simulink model "MassSpringDamperModel"  (R2026a)
settings: Solver=VariableStepAuto  StopTime=Inf  MaxStep=inf  RelTol=1e-6
values from neighbouring files (symbols this model uses):
  b = 1.0    [MassSpringDamperModelData.sldd]    (also in MassSpringDamperModelEventsData.sldd = 3.0)
  k = 100.0    [MassSpringDamperModelData.sldd]    (also in MassSpringDamperModelEventsData.sldd = 128.0)
  m = 10.0    [MassSpringDamperModelData.sldd]    (also in MassSpringDamperModelEventsData.sldd = 2.0)
  x0 = 0.5    [MassSpringDamperModelData.sldd]    (also in MassSpringDamperModelEventsData.sldd = 5.0)
libraries: simulink x1
Description:
  | The van der Pol Equation
  | 
  | This is a simulation of a nonlinear second order system.
settings Model: DataDictionary=MassSpringDamperModelData.sldd  ExtModeAutoUpdateStatusClock=off  Creator=The MathWorks, Inc.  LastModifiedBy=kdeeley
settings DataIOCC: ExternalInput=[]  InitialState=[]  TimeSaveName=t  OutputSaveName=y
settings OptimizationCC: BooleanDataType=off  InitFltsAndDblsToZero=on  BufferReusableBoundary=off
settings DebuggingCC: SaveWithParameterizedLinksMsg=none  SignalResolutionControl=TryResolveAllWithWarning  MultiTaskDSMMsg=warning  MultiTaskCondExecSysMsg=none  BusObjectLabelMismatch=none  PregeneratedLibrarySubsystemCodeDiagnostic=none
settings HardwareCC: ProdHWDeviceType=32-bit Generic  TargetUnknown=on
settings GRTTargetCC: TargetFcnLib=ansi_tfl_tmw.mat  CombineOutputUpdateFcns=off  GRTInterface=on

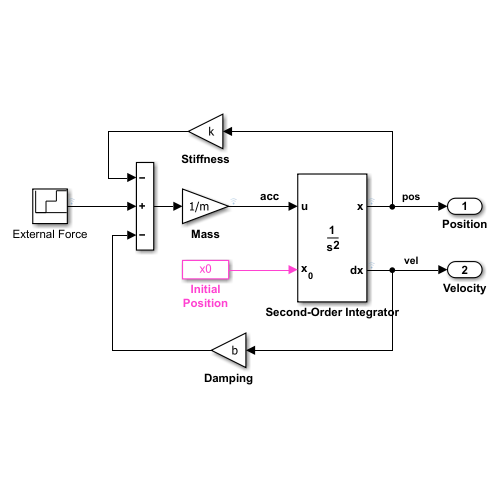
[thumbnail: Simulink's stored preview of the top-level diagram]
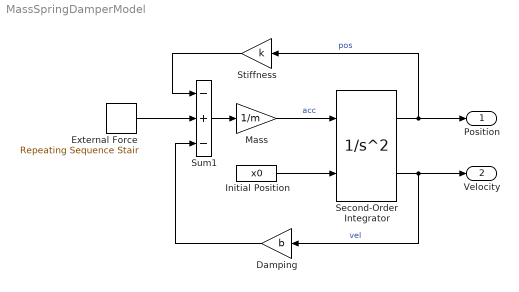
== system MassSpringDamperModel ==
  Damping : Gain  Gain=b
  External Force : simulink/Sources/Repeating Sequence Stair  OutValues=[0; 10; 20].'  tsamp=10  OutMin=[]  OutMax=[]  OutDataTypeStr=double  OutputDataTypeScalingMode=double  OutDataType=fixdt(0,8)  ConRadixGroup=Best Precision: Vector-wise  OutScaling=2^-12
  Initial Position : Constant  Value=x0
  Mass : Gain  Gain=1/m
  Second-Order Integrator : SecondOrderIntegrator  ICSourceX=external  StateNameX='pos'  StateNameDXDT='vel'  ReinitDXDTwhenXreachesSaturation=on
  Stiffness : Gain  Gain=k
  Sum1 : Sum  Inputs=-+-
  Position : Outport  VectorParamsAs1DForOutWhenUnconnected=off
  Velocity : Outport  Port=2  VectorParamsAs1DForOutWhenUnconnected=off
  wires:
  Sum1/1 -> Mass/1
  Mass/1 -> Second-Order Integrator/1  "acc"
  External Force/1 -> Sum1/2
  Second-Order Integrator/1 -> Stiffness/1, Position/1  "pos"
  Stiffness/1 -> Sum1/1
  Second-Order Integrator/2 -> Damping/1, Velocity/1  "vel"
  Initial Position/1 -> Second-Order Integrator/2
  Damping/1 -> Sum1/3
